simulink model "Simulink_21_10"  (R2020a)
settings: Solver=VariableStepAuto  StartTime=0.0  StopTime=45  RelTol=1e-3
libraries: cstblocks x10, simulink x2
settings Model: Creator=geral  LastModifiedBy=Sebas

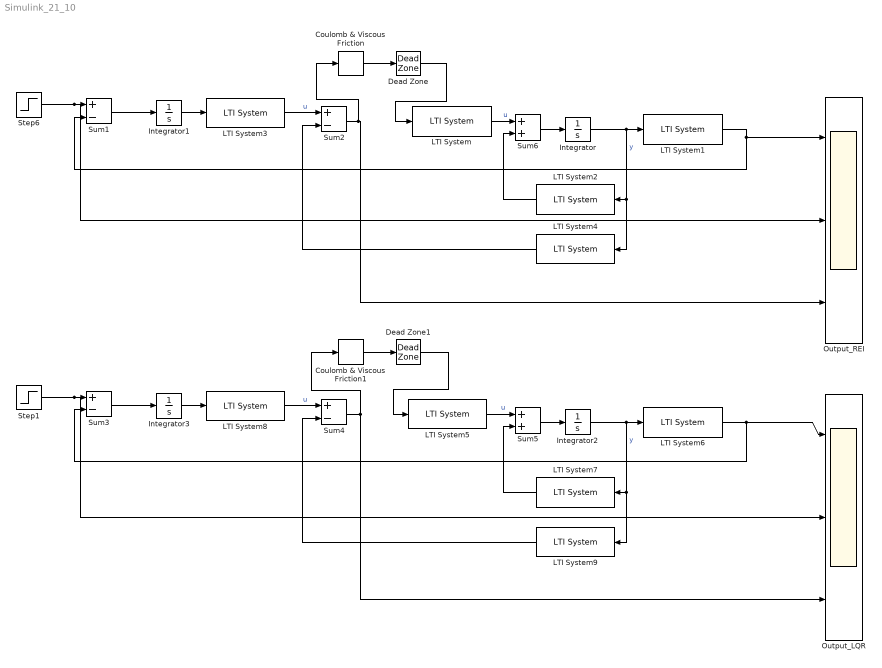
== system Simulink_21_10 ==
  Coulomb & Viscous Friction : simulink/Discontinuities/Coulomb & Viscous Friction  offset=[0.4]  gain=1
  Coulomb & Viscous Friction1 : simulink/Discontinuities/Coulomb & Viscous Friction  offset=[0.4]  gain=1
  Dead Zone : DeadZone  UpperValue=0.6  SaturateOnIntegerOverflow=on
  Dead Zone1 : DeadZone  UpperValue=0.6  SaturateOnIntegerOverflow=on
  Integrator{,1..3} (4 alike) : Integrator
  LTI System : cstblocks/LTI System  sys=Grua_ss.B  IC=[]
  LTI System1 : cstblocks/LTI System  sys=[1 0 0 0]  IC=[]
  LTI System2 : cstblocks/LTI System  sys=Grua_ss.A  IC=[]
  LTI System3 : cstblocks/LTI System  sys=Ki_REI  IC=[]
  LTI System4 : cstblocks/LTI System  sys=K_REI  IC=[]
  LTI System5 : cstblocks/LTI System  sys=Grua_ss.B  IC=[]
  LTI System6 : cstblocks/LTI System  sys=[1 0 0 0]  IC=[]
  LTI System7 : cstblocks/LTI System  sys=Grua_ss.A  IC=[]
  LTI System8 : cstblocks/LTI System  sys=Ki_LQR  IC=[]
  LTI System9 : cstblocks/LTI System  sys=K_LQR  IC=[]
  Output_LQR : Scope  NumInputPorts=3
  Output_REI : Scope  NumInputPorts=3
  Step1 : Step  Time=0.1  After=7.5  SampleTime=0
  Step6 : Step  Time=0.1  After=7.5  SampleTime=0
  Sum{1..4} (4 alike) : Sum  Inputs=+-
  Sum5 : Sum
  Sum6 : Sum
  wires:
  Sum6/1 -> Integrator/1
  LTI System/1 -> Sum6/1  "u"
  Integrator/1 -> LTI System1/1, LTI System4/1, LTI System2/1  "y"
  LTI System2/1 -> Sum6/2
  LTI System1/1 -> Sum1/2, Output_REI/1
  Step6/1 -> Output_REI/2, Sum1/1
  Sum1/1 -> Integrator1/1
  Integrator1/1 -> LTI System3/1
  LTI System3/1 -> Sum2/1  "u"
  Sum2/1 -> Coulomb & Viscous Friction/1, Output_REI/3
  LTI System4/1 -> Sum2/2
  LTI System5/1 -> Sum5/1  "u"
  Integrator3/1 -> LTI System8/1
  LTI System7/1 -> Sum5/2
  LTI System8/1 -> Sum4/1  "u"
  Step1/1 -> Output_LQR/2, Sum3/1
  LTI System6/1 -> Sum3/2, Output_LQR/1
  Sum3/1 -> Integrator3/1
  Integrator2/1 -> LTI System6/1, LTI System9/1, LTI System7/1  "y"
  Sum5/1 -> Integrator2/1
  LTI System9/1 -> Sum4/2
  Coulomb & Viscous Friction/1 -> Dead Zone/1
  Dead Zone/1 -> LTI System/1
  Dead Zone1/1 -> LTI System5/1
  Coulomb & Viscous Friction1/1 -> Dead Zone1/1
  Sum4/1 -> Output_LQR/3, Coulomb & Viscous Friction1/1
